simulink model "MPC"  (R2023b)
settings: Solver=FixedStepAuto  StartTime=0.0  StopTime=20  FixedStep=0.01  RelTol=1e-3
values from neighbouring files (symbols this model uses):
  D = zeros(3)    [LMPC.m]
libraries: vehdynlibviscommon x1, autolibshared x1, mpclib x1, robotcorelib x1, sim3dlib x1, sim3dautolib x1
settings Model: Creator=Arash  LastModifiedBy=Arash

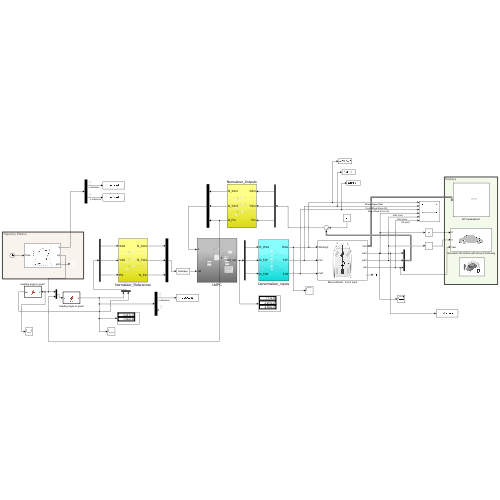
[thumbnail: Simulink's stored preview of the top-level diagram]
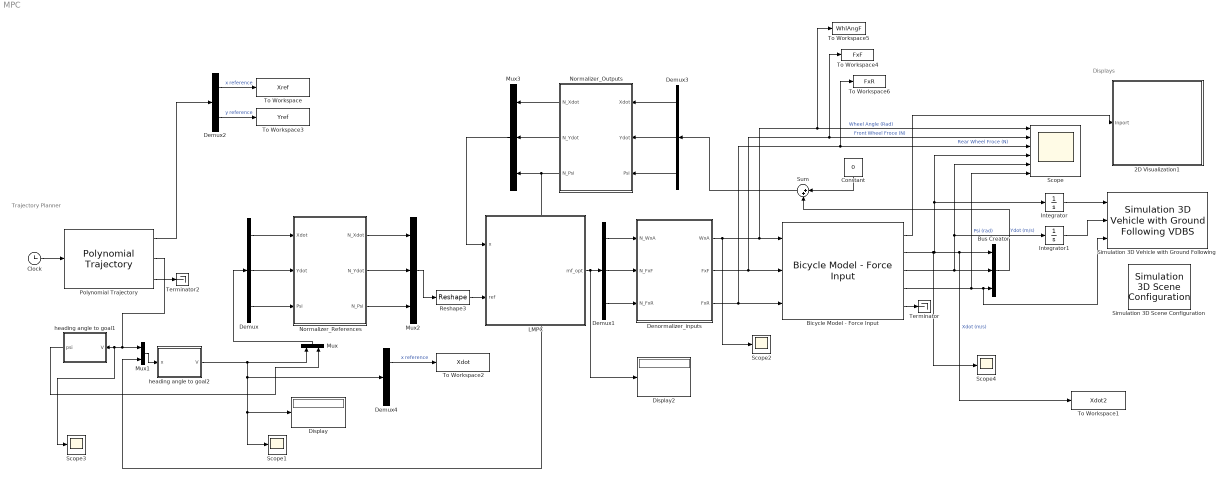
== system MPC ==
  note: Trajectory Planner
  note: Displays
  2D Visualization1 : Subsystem
      mask Display: image("visualization.JPG");
  Bicycle Model - Force Input : autolibshared/Bicycle Model - Force Input  trackMode=Single (bicycle)  inputMode=External longitudinal forces  frontSteerMode=on  rearSteerMode=off  windMode=off  muMode=off  extFMode=off  extMMode=off  aMode=3  NF=2  NR=2  m=2000  a=1.4  b=1.6  h=0.35  X_o=0  xdot_o=0  CalphaMode=off  sigmaMode=on  w=[1.4,1.4]  Cy_f=12e3  Cy_r=11e3  sigma_f=.1  sigma_r=.1  alpha_f_brk=[-.1 .1]  Cy_f_data=[-9e3 9e3]  alpha_r_brk=[-.1 .1]  Cy_r_data=[-9e3 9e3]  Y_o=0  ydot_o=0  Izz=4000  psi_o=0  r_o=0  Af=2  Cd=.3  Cl=.1  Cpm=.1  beta_w=[0 0.01:0.01:0.3]  Cs=[0 0.01:0.01:0.3]  Cym=[0 1e-6:0.01:0.3]  Pabs=101325  Tair=273  g=9.81  mu=1  xdot_tol=.01  Fznom=5000  Fxtire_sat=1e6  Fytire_sat=1e6  longOff=0  latOff=0  vertOff=0
      settings: LibrarySourceBlock=drivingscenarioandsensors/Bicycle Model - Force Input
  Bus Creator : BusCreator  Inputs=3
  Clock : Clock
      settings: Decimation=19
  Constant : Constant  Value=0
  Demux : Demux  Outputs=3
  Demux1 : Demux  Outputs=3
  Demux2 : Demux  Outputs=2
  Demux3 : Demux  Outputs=3
  Demux4 : Demux  Outputs=2
  Denormalizer_inputs : Subsystem
  Display : Display
  Display2 : Display
  Integrator : Integrator
  Integrator1 : Integrator
  LMPC : Subsystem
  Mux : Mux  Inputs=2
  Mux1 : Mux  Inputs=2
  Mux2 : Mux  Inputs=3
  Mux3 : Mux  Inputs=3
  Normalizer_Outputs : Subsystem
  Normalizer_References : Subsystem
  Polynomial Trajectory : robotcorelib/Polynomial Trajectory  WaypointSource=Internal  Waypoints=[0,10; 0,0]  TimePoints=[0,20]  TimeInterval=[ 1, 4 ]  Method=Cubic Polynomial  ParameterSource=Internal  VelocityBoundaryCondition=zeros( 2, 2)  AccelerationBoundaryCondition=zeros( 2, 5 )  SimulateUsing=Interpreted execution
  Reshape3 : Reshape  OutputDimensionality=Customize  OutputDimensions=[1,3]
  Scope : Scope  NumInputPorts=6
  Scope{1..4} (4 alike) : Scope
  Simulation 3D Scene Configuration : sim3dlib/Simulation 3D Scene Configuration  Priority=0  ProjectFormat=Default Scenes  SceneDesc=Straight road  ProjectName=C:\Program Files\MATLAB\R2023b\toolbox\shared\sim3d_projects\automotive_project_windows\UE\WindowsNoEditor\VehicleSimulation.exe  ScenePath=/Game/Maps/HwStrght  EnableOpenDRIVE=off  vehTagList={'Scene Origin'}  vehTag=Scene Origin  FreeCameraInitialTranslation=[0, 0, 0]  FreeCameraDefaultInitialTranslation=[-6, 0, 2]  FreeCameraInitialRotation=[0, 0, 0]  FreeCameraDefaultInitialRotation=[0, -15, 0]  OpVisEn=off  Ts=0.1  EnableWindow=on  EnableRemoteAccess=off  EnableWeather=off  SunAltitude=40.0  SunAzimuth=90  clouds=10  wind=1  fog=0  rain=0  EnableGeospatial=off  OriginHeight=200  OriginLatitude=40.744652  OriginLongitude=-73.988864  MapStyle=Aerial  AdditionalAssetIDs=[]  UseAdvancedSunSky=off  SolarTime=11  TimeZone=-5  Day=21  Month=9  Year=2022  UseDaylightSavingTime=on  DSTStartDay=10  DSTStartMonth=3  DSTEndDay=3  DSTEndMonth=11  DSTSwitchHour=2  sensorTag=MainCamera1  sensorId=1  sensorName=MainCamera1  mountLoc=Origin  offsetFlag=off  tmountOffset=[0, 0, 0]  rmountOffset=[0, 0, 0]  HorizontalResolution=1280  VerticalResolution=720  HorizontalFOV=60  mountPoint=[0 0 0]  mountOrientation=[0 0 0]  aMode=aMode  ID=1  GeoTrigger=Inactive
  Simulation 3D Vehicle with Ground Following : sim3dautolib/Simulation 3D Vehicle with Ground Following VDBS  Priority=-1  PassVehMesh=Hatchback  MeshPath=/MathWorksSimulation/Vehicles/Muscle/Meshes/SK_MuscleCar.SK_MuscleCar  TrackWidth=1.9  WheelBase=3  WheelRadius=0.35  VehColor=Green  InitialPos=[0,0,0]  InitialRot=[0, 0, 0]  ActorName=SimulinkVehicle1  VehLightsControl=off  HeadlightColor=[ 1, 1, 1 ]  HighBeamIntensity=100000  LowBeamIntensity=60000  HighBeamConeAngle=1.22  LowBeamConeAngle=1.22  LeftHeadlightOrientation=[ 0, 0 ]  RightHeadlightOrientation=[ 0, 0 ]  BrakelightIntensity=200  ReverselightIntensity=500  SignallightIntensity=500  SignallightPeriod=1  SignalPulseWidth=50  SampleTime=-1  ActorType=SimulinkVehicle  ID=1  aMode=2  ActorTag=SimulinkVehicle1  CoordinateScheme=SAE
      settings: LibrarySourceBlock=vehdynlibsim3d/Simulation 3D Vehicle with Ground Following
  Sum : Sum  Inputs=|++
  Terminator : Terminator
  Terminator2 : Terminator
  To Workspace : ToWorkspace  VariableName=Xref  SampleTime=-1
      settings: Save2DSignal=2-D array (concatenate along first dimension)
  To Workspace1 : ToWorkspace  VariableName=Xdot2  SaveFormat=Timeseries  SampleTime=-1
  To Workspace2 : ToWorkspace  VariableName=Xdot  SaveFormat=Timeseries  SampleTime=-1
  To Workspace3 : ToWorkspace  VariableName=Yref  SampleTime=-1
      settings: Save2DSignal=2-D array (concatenate along first dimension)
  To Workspace4 : ToWorkspace  VariableName=FxF  SaveFormat=Timeseries  SampleTime=0.1
  To Workspace5 : ToWorkspace  VariableName=WhlAngF  SaveFormat=Timeseries  SampleTime=0.1
  To Workspace6 : ToWorkspace  VariableName=FxR  SaveFormat=Timeseries  SampleTime=0.1
  heading angle to goal1 : MATLAB Function  TreatAsAtomicUnit=on
  heading angle to goal2 : MATLAB Function  TreatAsAtomicUnit=on
  wires:
  LMPC/1(mf_opt) -> Demux1/1, Display2/1
  Polynomial Trajectory/3 -> Terminator2/1
  Polynomial Trajectory/1 -> Demux2/1
  Clock/1 -> Polynomial Trajectory/1
  Demux2/1 -> To Workspace/1  "x reference"
  Demux2/2 -> To Workspace3/1  "y reference"
  Bicycle Model - Force Input/2 -> Scope4/1, Scope/4, Integrator/1, To Workspace1/1, Bus Creator/1  "Xdot (m/s)"
  Bicycle Model - Force Input/3 -> Scope/5, Integrator1/1, Bus Creator/2  "Ydot (m/s)"
  Bicycle Model - Force Input/4 -> Simulation 3D Vehicle with Ground Following/3, Bus Creator/3, Scope/6  "Psi (rad)"
  Bus Creator/1 -> Sum/2
  Bicycle Model - Force Input/1 -> 2D Visualization1/1(Inport)
  Integrator/1 -> Simulation 3D Vehicle with Ground Following/1
  Integrator1/1 -> Simulation 3D Vehicle with Ground Following/2
  Polynomial Trajectory/2 -> Scope3/1, heading angle to goal1/1(V), Mux1/1
  Mux1/1 -> heading angle to goal2/1(x)
  heading angle to goal2/1(V) -> Scope1/1, Display/1, Demux4/1, Mux/1
  Normalizer_References/2(N_Ydot) -> Mux2/2
  Demux/1 -> Normalizer_References/1(Xdot)
  Mux2/1 -> Reshape3/1
  Normalizer_References/1(N_Xdot) -> Mux2/1
  Mux/1 -> Demux/1
  Demux/2 -> Normalizer_References/2(Ydot)
  Demux/3 -> Normalizer_References/3(Psi)
  Normalizer_References/3(N_Psi) -> Mux2/3
  Reshape3/1 -> LMPC/2(ref)
  Denormalizer_inputs/3(FxR) -> To Workspace6/1, Scope/3, Bicycle Model - Force Input/3  "Rear Wheel Froce (N)"
  Demux1/3 -> Denormalizer_inputs/3(N_FxR)
  Denormalizer_inputs/2(FxF) -> To Workspace4/1, Scope/2, Bicycle Model - Force Input/2  "Front Wheel Froce (N)"
  Demux1/2 -> Denormalizer_inputs/2(N_FxF)
  Demux1/1 -> Denormalizer_inputs/1(N_WxA)
  Denormalizer_inputs/1(WxA) -> Scope2/1, To Workspace5/1, Scope/1, Bicycle Model - Force Input/1  "Wheel Angle (Rad)"
  Demux3/2 -> Normalizer_Outputs/2(Ydot)
  Normalizer_Outputs/3(N_Psi) -> Mux3/3, Mux1/2
  Normalizer_Outputs/1(N_Xdot) -> Mux3/1
  Demux3/3 -> Normalizer_Outputs/3(Psi)
  Demux3/1 -> Normalizer_Outputs/1(Xdot)
  Normalizer_Outputs/2(N_Ydot) -> Mux3/2
  Mux3/1 -> LMPC/1(x)
  Bicycle Model - Force Input/5 -> Terminator/1
  heading angle to goal1/1(psi) -> Mux/2
  Demux4/1 -> To Workspace2/1  "x reference"
  Constant/1 -> Sum/1
  Sum/1 -> Demux3/1

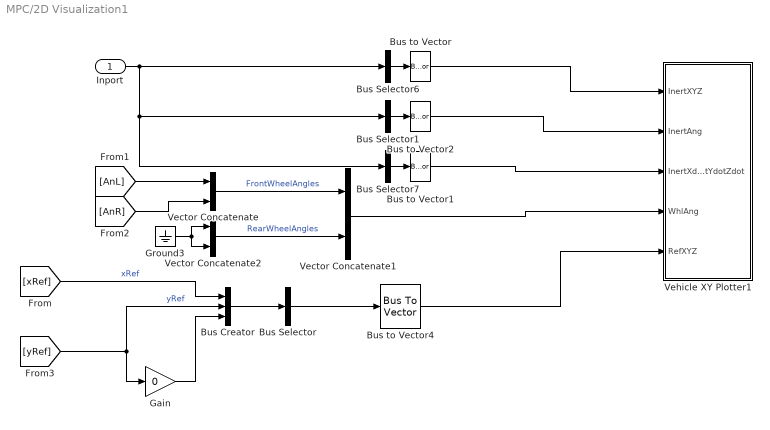
== system MPC/2D Visualization1 ==
  Inport : Inport
  Bus Creator : BusCreator  Inputs=3
  Bus Selector : BusSelector  OutputSignals=xRef,yRef,signal3  OutputAsBus=on
  Bus Selector1 : BusSelector  OutputSignals=InertFrm.Cg.Ang.phi,InertFrm.Cg.Ang.theta,InertFrm.Cg.Ang.psi  OutputAsBus=on
  Bus Selector6 : BusSelector  OutputSignals=InertFrm.Geom.Disp.X,InertFrm.Geom.Disp.Y,InertFrm.Geom.Disp.Z  OutputAsBus=on
  Bus Selector7 : BusSelector  OutputSignals=InertFrm.Geom.Vel.Xdot,InertFrm.Geom.Vel.Ydot,InertFrm.Geom.Vel.Zdot  OutputAsBus=on
  Bus to Vector{,1..2,4} (4 alike) : BusToVector
  Gain : Gain  Gain=0
  Ground3 : Ground
  Vector Concatenate : Concatenate
  Vector Concatenate1 : Concatenate
  Vector Concatenate2 : Concatenate
  Vehicle XY Plotter1 : Subsystem  mask(Vehicle XY Plotter){extRef=on, extStats=off, extTireF=off, a=2, b=2, w=2, figBorder=10, bufferSize=1024, velNorm=5, tireFNorm=1000, pltDT=0.2}
      mask prompts: extRef "Plot path reference, extRef"; extStats "Display speed, RPM and Gear"; extTireF "Display tire forces"; a "Distance to front axle from CG, a [m]:"; b "Distance to rear axle from CG, b [m]:"; w "Track width, w [m]:"; figBorder "Distance to figure borders, figBorder [m]:"; bufferSize "Path buffer sampe size, bufferSize []:"; velNorm "Velocity vector scaling, velNorm [m*s/m]:"; tireFNorm "Tire force vector scaling, tireFNorm [m/N]:"; pltDT "Plot update rate, pltDT [s]:"
      mask help:
      | This block will display a MATLAB figure which indicates the vehicle path, current position and heading velocity.
      | An optional path reference is also provided.
      mask init:
      | block = gcb;
      | if autoblkschecksimstopped(block)
      |     ParamNames = {'extRef';'extStats';'extTireF';'extTireF'};
      |     PortNames = {'RefXYZ';'Stats';'TireFx';'TireFy'};
      |     for idx=1:length(PortNames)
      |         InportOption  = {'built-in/Ground', [PortNames{idx}, ' Ground'];...
      |             'built-in/Inport',PortNames{idx}};
      |         if ~strcmp(get_param(block,ParamNames{idx}),'on')
      |             NewBlkHdl = autoblksreplaceblock(block, InportOption, 1);
      |             set_param(NewBlkHdl, 'ShowName', 'off');
      |         else
      |             autoblksreplaceblock(block, InportOption, 2);
      |         end
      |     end
      |     InportNames = {'InertXYZ';'InertAng';'InertXdotYdotZdot';'WhlAng';'RefXYZ';'Stats';'TireFx';'TireFy'};
      |     FoundNames = get_param(find_system(block, 'LookUnderMasks', 'all', 'SearchDepth', 1, 'FollowLinks', 'on', 'BlockType', 'Inport'), 'Name');
      |     [~,PortI] = intersect(InportNames, FoundNames);
      |     PortI = sort(PortI);
      |     for idx = 1:length(PortI)
      |         set_param([block, '/', InportNames{PortI(idx)}], 'Port', num2str(idx));
      |     end
      | end
      mask TypeOptions a: Vehicle XY Plotter/a
      mask TypeOptions b: Vehicle XY Plotter/b
      mask TypeOptions w: Vehicle XY Plotter/w
      mask TypeOptions figBorder: Vehicle XY Plotter/figBorder
      mask TypeOptions bufferSize: Vehicle XY Plotter/bufferSize
      mask TypeOptions velNorm: Vehicle XY Plotter/velNorm
      mask TypeOptions tireFNorm: Vehicle XY Plotter/tireFNorm
      mask DialogControl Container3 Prompt: Plot and Display Options
  wires:
  Bus Creator/1 -> Bus Selector/1
  [xRef] -> Bus Creator/1  "xRef"
  Gain/1 -> Bus Creator/3
  [yRef] -> Gain/1, Bus Creator/2  "yRef"
  Bus Selector/1 -> Bus to Vector4/1
  Bus to Vector4/1 -> Vehicle XY Plotter1/5(RefXYZ)
  Inport/1 -> Bus Selector6/1, Bus Selector1/1, Bus Selector7/1
  [AnR] -> Vector Concatenate/2
  Bus Selector1/1 -> Bus to Vector2/1
  Bus to Vector2/1 -> Vehicle XY Plotter1/2(InertAng)
  Bus to Vector/1 -> Vehicle XY Plotter1/1(InertXYZ)
  Bus to Vector1/1 -> Vehicle XY Plotter1/3(InertXdotYdotZdot)
  Bus Selector7/1 -> Bus to Vector1/1
  Vector Concatenate2/1 -> Vector Concatenate1/2  "RearWheelAngles"
  [AnL] -> Vector Concatenate/1
  Vector Concatenate/1 -> Vector Concatenate1/1  "FrontWheelAngles"
  Bus Selector6/1 -> Bus to Vector/1
  Ground3/1 -> Vector Concatenate2/2, Vector Concatenate2/1
  Vector Concatenate1/1 -> Vehicle XY Plotter1/4(WhlAng)

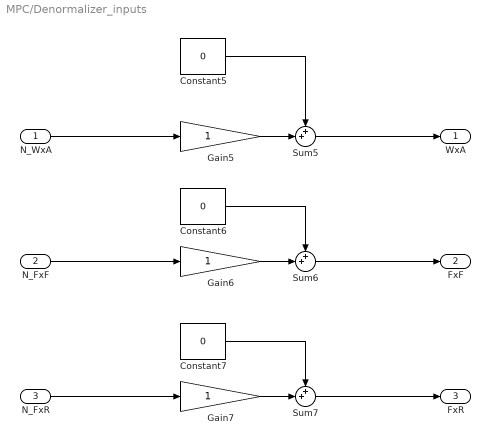
== system MPC/Denormalizer_inputs ==
  N_WxA : Inport
  N_FxF : Inport  Port=2
  N_FxR : Inport  Port=3
  Constant5 : Constant  Value=0
  Constant6 : Constant  Value=0
  Constant7 : Constant  Value=0
  Gain5 : Gain
  Gain6 : Gain
  Gain7 : Gain
  Sum5 : Sum  Inputs=++|
  Sum6 : Sum  Inputs=++|
  Sum7 : Sum  Inputs=++|
  WxA : Outport
  FxF : Outport  Port=2
  FxR : Outport  Port=3
  wires:
  Sum6/1 -> FxF/1
  Gain7/1 -> Sum7/2
  Gain5/1 -> Sum5/2
  Constant7/1 -> Sum7/1
  Gain6/1 -> Sum6/2
  Sum5/1 -> WxA/1
  Constant5/1 -> Sum5/1
  Constant6/1 -> Sum6/1
  Sum7/1 -> FxR/1
  N_FxR/1 -> Gain7/1
  N_WxA/1 -> Gain5/1
  N_FxF/1 -> Gain6/1

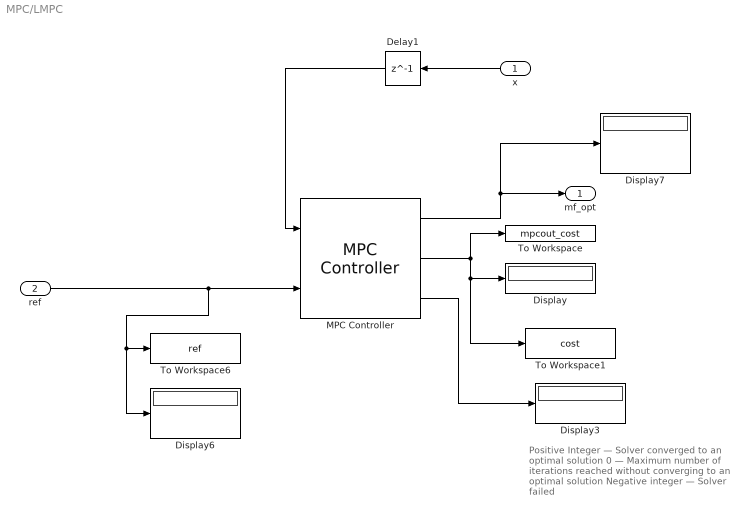
== system MPC/LMPC ==
  note: Positive Integer — Solver converged to an optimal solution
      | 0 — Maximum number of iterations reached without converging to an optimal solution
      | Negative integer — Solver failed
  x : Inport
  ref : Inport  Port=2
  Delay1 : Delay  DelayLength=1  InitialCondition=0
  Display{,3,6..7} (4 alike) : Display
  MPC Controller : mpclib/MPC Controller  SCDEnableBlockLinearizationSpecification=on  mpcobj=mpcobj  is_multiple=0  enable_value=0  return_u0=off  updateMPCinCallerWorkspace=on  md_inport=off  mv_inport=off  uref_inport=off  return_cost=on  return_mvseq=off  return_qpstatus=on  return_xseq=off  return_state=off  return_ovseq=off  state_inport=off  umin_inport=off  umax_inport=off  ymin_inport=off  ymax_inport=off  cc_inport=off  ywt_inport=off  uwt_inport=off  duwt_inport=off  rhoeps_inport=off  pm_inport=off  MaximumP=10  HorizonChoice=FixedHorizon  n_ts=0.1  n_p=75  n_mv=3  n_md=0  n_ud=0  n_mo=3  n_uo=0  BlockDataType=double  SampleTimeInherited=off  switch_inport=off
  To Workspace : ToWorkspace  VariableName=mpcout_cost  SaveFormat=Timeseries  SampleTime=-1
  To Workspace1 : ToWorkspace  VariableName=cost  SaveFormat=Timeseries  SampleTime=-1
  To Workspace6 : ToWorkspace  VariableName=ref  SaveFormat=Timeseries  SampleTime=-1
  mf_opt : Outport
  wires:
  MPC Controller/1 -> Display7/1, mf_opt/1
  x/1 -> Delay1/1
  ref/1 -> MPC Controller/2, Display6/1, To Workspace6/1
  MPC Controller/2 -> To Workspace1/1, Display/1, To Workspace/1
  MPC Controller/3 -> Display3/1
  Delay1/1 -> MPC Controller/1

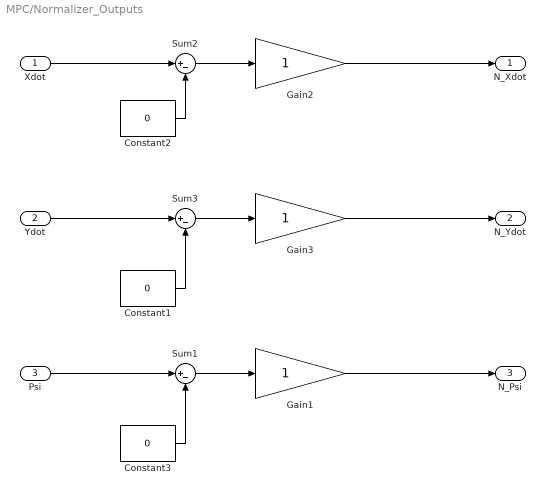
== system MPC/Normalizer_Outputs ==
  Xdot : Inport
  Ydot : Inport  Port=2
  Psi : Inport  Port=3
  Constant1 : Constant  Value=0
  Constant2 : Constant  Value=0
  Constant3 : Constant  Value=0
  Gain1 : Gain
  Gain2 : Gain
  Gain3 : Gain
  Sum1 : Sum  Inputs=|+-
  Sum2 : Sum  Inputs=|+-
  Sum3 : Sum  Inputs=|+-
  N_Xdot : Outport
  N_Ydot : Outport  Port=2
  N_Psi : Outport  Port=3
  wires:
  Gain2/1 -> N_Xdot/1
  Sum3/1 -> Gain3/1
  Constant2/1 -> Sum2/2
  Gain3/1 -> N_Ydot/1
  Constant1/1 -> Sum3/2
  Sum2/1 -> Gain2/1
  Xdot/1 -> Sum2/1
  Ydot/1 -> Sum3/1
  Sum1/1 -> Gain1/1
  Gain1/1 -> N_Psi/1
  Constant3/1 -> Sum1/2
  Psi/1 -> Sum1/1

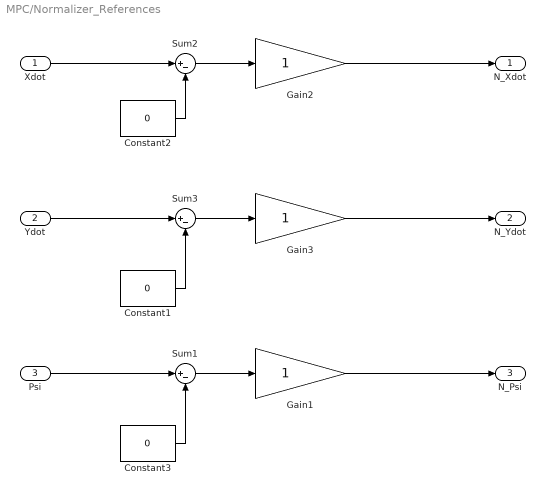
== system MPC/Normalizer_References ==
  Xdot : Inport
  Ydot : Inport  Port=2
  Psi : Inport  Port=3
  Constant1 : Constant  Value=0
  Constant2 : Constant  Value=0
  Constant3 : Constant  Value=0
  Gain1 : Gain
  Gain2 : Gain
  Gain3 : Gain
  Sum1 : Sum  Inputs=|+-
  Sum2 : Sum  Inputs=|+-
  Sum3 : Sum  Inputs=|+-
  N_Xdot : Outport
  N_Ydot : Outport  Port=2
  N_Psi : Outport  Port=3
  wires:
  Gain2/1 -> N_Xdot/1
  Sum3/1 -> Gain3/1
  Constant2/1 -> Sum2/2
  Gain3/1 -> N_Ydot/1
  Constant1/1 -> Sum3/2
  Sum2/1 -> Gain2/1
  Xdot/1 -> Sum2/1
  Ydot/1 -> Sum3/1
  Sum1/1 -> Gain1/1
  Gain1/1 -> N_Psi/1
  Constant3/1 -> Sum1/2
  Psi/1 -> Sum1/1

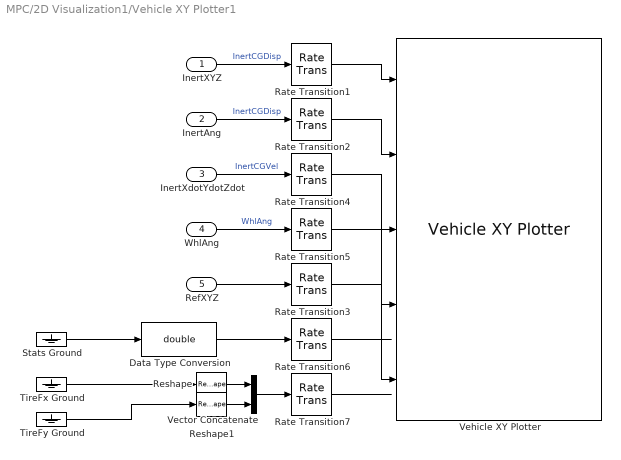
== system MPC/2D Visualization1/Vehicle XY Plotter1 ==
  InertXYZ : Inport
  InertAng : Inport  Port=2
  InertXdotYdotZdot : Inport  Port=3
  WhlAng : Inport  Port=4
  RefXYZ : Inport  Port=5
  Data Type Conversion : DataTypeConversion  OutDataTypeStr=double  SaturateOnIntegerOverflow=off  RndMeth=Floor
  Rate Transition{1..7} (7 alike) : RateTransition  Deterministic=off  OutPortSampleTime=pltDT
  Reshape : Reshape  OutputDimensionality=Row vector (2-D)
  Reshape1 : Reshape  OutputDimensionality=Row vector (2-D)
  Stats Ground : Ground
  TireFx Ground : Ground
  TireFy Ground : Ground
  Vector Concatenate : Concatenate  Mode=Multidimensional array
  Vehicle XY Plotter : vehdynlibviscommon/Vehicle XY Plotter  w=w  a=a  b=b  figBorder=figBorder  bufferSize=bufferSize  extStats=off  extTireF=off
  wires:
  TireFy Ground/1 -> Reshape1/1
  TireFx Ground/1 -> Reshape/1
  Stats Ground/1 -> Data Type Conversion/1
  InertAng/1 -> Rate Transition2/1  "InertCGDisp"
  InertXdotYdotZdot/1 -> Rate Transition4/1  "InertCGVel"
  InertXYZ/1 -> Rate Transition1/1  "InertCGDisp"
  WhlAng/1 -> Rate Transition5/1  "WhlAng"
  Rate Transition3/1 -> Vehicle XY Plotter/5
  Rate Transition1/1 -> Vehicle XY Plotter/1
  Rate Transition2/1 -> Vehicle XY Plotter/2
  Rate Transition4/1 -> Vehicle XY Plotter/3
  Rate Transition5/1 -> Vehicle XY Plotter/4
  Rate Transition6/1 -> ?
  Data Type Conversion/1 -> Rate Transition6/1
  Rate Transition7/1 -> ?
  RefXYZ/1 -> Rate Transition3/1
  Reshape/1 -> Vector Concatenate/1
  Reshape1/1 -> Vector Concatenate/2
  Vector Concatenate/1 -> Rate Transition7/1

== matlab function MPC/heading angle to goal2 ==
  data: x input; V output
function V = fcn(x)


V = [cos(x(3)) sin(x(3));
    -sin(x(3)) cos(x(3))]*[x(1); x(2)];

== matlab function MPC/heading angle to goal1 ==
  data: V input; psi output
function psi = fcn(V)

v1 =V(1);
v2 =V(2);
psi = atan2(v2,v1);
